simulink model "Continuous5_2018a"  (R2018a)
settings: Solver=VariableStepAuto  StartTime=0.0  StopTime=2  FixedStep=0.1  RelTol=1e-3  EnableMultiTasking=on
settings Model: Creator=BEAR  LastModifiedBy=bzhan
settings SolverCC: AutoInsertRateTranBlk=on
settings DataIOCC: LimitDataPoints=on
settings OptimizationCC: LifeSpan=inf
settings DebuggingCC: AllowSymbolicDim=off  SFUnexpectedBacktrackingDiag=warning  SFNoUnconditionalDefaultTransitionDiag=warning  SFExecutionAtInitializationDiag=none
settings CodeAppCC: StateflowObjectComments=on
settings GRTTargetCC: TargetLangStandard=C89/C90 (ANSI)
settings ConfigComp: CovMetricSettings=dw  CovHtmlReporting=on  CovSaveCumulativeToWorkspaceVar=on  CovSaveSingleToWorkspaceVar=on  CovShowResultsExplorer=off  CovExternalEMLEnable=off  CovSFcnEnable=off

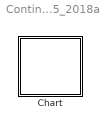
== system Continuous5_2018a ==
  Chart : Stateflow chart  TreatAsAtomicUnit=on

== stateflow chart Continuous5_2018a/Chart ==
  settings: updateMethod=CONTINUOUS
  state A
    en: f("enA")
    du: x_dot=1;
    ex: f("exA")
    state A1
      en: f("enA1")
    state A2
      en: f("enA2")
    (default) -> A1
    A1 -> A2 : [x>=1]
  state B
    en: f("enB");
    x=0;
    du: x_dot=1;
  (default) -> A : {x=0;}
  A -> B : [x>=2]
  B -> B : [x>=1]
  data: s function_input; x local double
  data x settings: updateMethod=SF_CONTINUOUS_TIME_DATA
  function f(s):
    | function f(s)
    |   fprintf(s+"\n");
